simulink model "rtwdemo_symbols"  (Simulink 7.6)
settings: Solver=FixedStepDiscrete  StartTime=0.0  StopTime=1  FixedStep=0.001  RelTol=1e-3
libraries: rtwdemowidgets x1
Description:
  | Identifier Naming Rules
settings Model: Creator=The MathWorks Inc.  ExtModeAutoUpdateStatusClock=off
settings MATStruct: SampleTime=0.001  Offset=0  Priority=[20.0]
settings DataIOCC: SaveOutput=off  SaveTime=off
settings OptimizationCC: InlineParams=on  InlineInvariantSignals=on  PassReuseOutputArgsAs=Individual arguments  StateBitsets=on  DataBitsets=on  UseTempVars=on  ZeroExternalMemoryAtStartup=off  ZeroInternalMemoryAtStartup=off  NoFixptDivByZeroProtection=on  EfficientFloat2IntCast=on  EfficientMapNaN2IntZero=off  OptimizeModelRefInitCode=on  LifeSpan=1  BufferReusableBoundary=off
settings DebuggingCC: CheckExecutionContextPreStartOutputMsg=on  CheckExecutionContextRuntimeOutputMsg=on  SigSpecEnsureSampleTimeMsg=none  StrictBusMsg=ErrorOnBusTreatedAsVector
settings HardwareCC: ProdIntDivRoundTo=Zero  ProdEndianess=LittleEndian  ProdHWDeviceType=Generic->32-bit Embedded Processor  TargetHWDeviceType=Generic->32-bit Embedded Processor
settings SFSimCC: SimParseCustomCode=off
settings RTWCC: SystemTargetFile=ert.tlc  TemplateMakefile=ert_default_tmf  Description=Real-Time Workshop Embedded Coder (no auto configuration)  GenerateReport=on  RTWVerbose=off  ProcessScript=ert_make_rtw_hook  IncludeHyperlinkInReport=on  LaunchReport=on
settings CodeAppCC: ForceParamTrailComments=on  IgnoreCustomStorageClasses=off  IgnoreTestpoints=on  MaxIdLength=40  SimulinkDataObjDesc=on  CustomSymbolStrMacro=$N$M  InsertBlockDesc=on
settings ERTTargetCC: TargetFcnLib=ansi_tfl_tmw.mat  MultiwordLength=2048  GenerateSampleERTMain=on  IncludeMdlTerminateFcn=off  SupportNonFinite=off  SupportComplex=off  InlinedParameterPlacement=NonHierarchical  ERTCustomFileTemplate=example_file_process.tlc  ConvertIfToSwitch=off

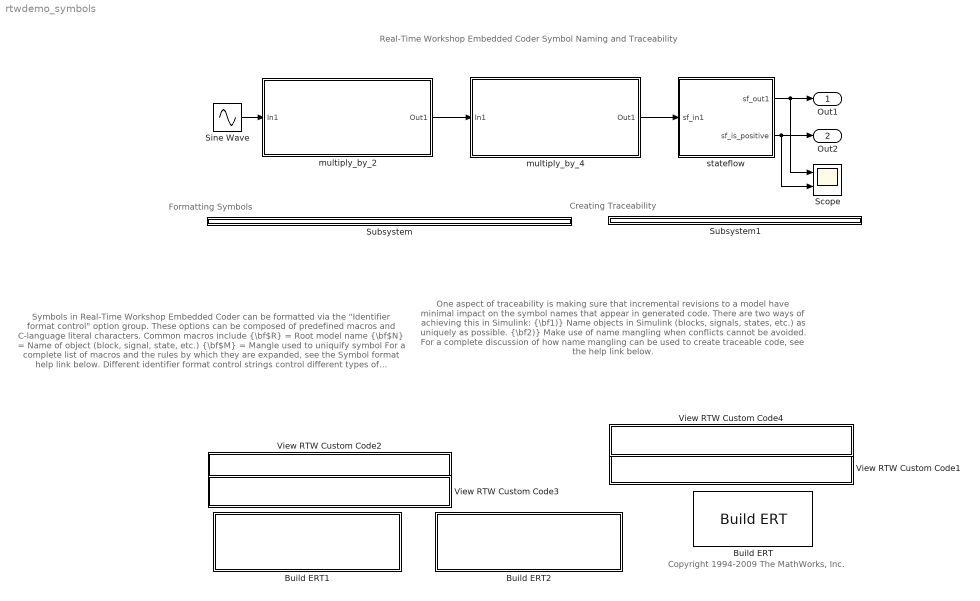
== system rtwdemo_symbols ==
  note: Real-Time Workshop Embedded Coder
      | Symbol Naming and Traceability
  note: Formatting Symbols
  note: Creating Traceability
  note: Symbols in Real-Time Workshop Embedded Coder can be formatted
      | via the "Identifier format control" option group. These options can be
      | composed of predefined macros and C-language literal characters.
      |
      | Common macros include
      |    {\bf$R} = Root model name
      |    {\bf$N} = Name of object (block, signal, state, etc.)
      |    {\bf$M} = Mangle used to uniquify symbol
      |
      | For a complete list of macros and the rules by which they are
      | expanded, see the Symbol format help link below.
      |
      | Different identifier format control strings control different types of identifiers.
      | Double-click the yellow buttons at the bottom to modify the format
      | control strings for global variable names and global type names. Double-
      | click the blue button to generate and inspect code for the change.
  note: One aspect of traceability is making sure that
      | incremental revisions to a model have minimal
      | impact on the symbol names that appear in
      | generated code.  There are two ways of
      | achieving this in Simulink:
      |
      |   {\bf1)} Name objects in Simulink (blocks, signals,
      |        states, etc.) as uniquely as possible.
      |   {\bf2)} Make use of name mangling when conflicts
      |        cannot be avoided.
      |
      | For a complete discussion of how name mangling
      | can be used to create traceable code, see the help
      | link below.
  note: Copyright 1994-2009 The MathWorks, Inc.
  Build ERT : rtwdemowidgets/Build ERT  SystemSampleTime=-1  attrib_overrides={'CustomSymbolStrGlobalVar', 'CustomSymbolStrType','CustomSymbolStrField','CustomSymbolStrFcn','CustomSymbolStrBlkIO','CustomSymbolStrTmpVar','CustomSymbolStrMacro'}
  Build ERT1 : Subsystem  mask{sfs=$R$N$M}
      mask prompts: sfs "symbol format string"
      mask help: Enter the attributes of the configuration set that you want preserved. Otherwise, the default configuration script will override your current settings.
      mask init:
      | if ~isempty(findstr(sfs, '$R'))
      |     dispstr = ['Global variable names\n', ...
      |             'contain model name.\n'];
      | else
      |     dispstr = ['Global variable names do\n',...
      |         'not contain model name.\n'];
      | end
      settings: OpenFcn=|
      | sfs = get_param(bdroot, 'CustomSymbolStrGlobalVar');
      | if strcmp(sfs, '$R$N$M')
      |   sfs = '$N$M';
      | else
      |   sfs = '$R$N$M';
      | end
      | set_param(bdroot, 'CustomSymbolStrGlobalVar', sfs);
      | set_param(gcbh, 'sfs', sfs);  clear sfs;
      mask Display:
      | disp([dispstr,...
      | 	  '(double-click to toggle)'])
  Build ERT2 : Subsystem  mask{sfs=$N$R$M}
      mask prompts: sfs "symbol format string"
      mask help: Enter the attributes of the configuration set that you want preserved. Otherwise, the default configuration script will override your current settings.
      mask init:
      | if ~isempty(findstr(sfs, '$R'))
      |     dispstr = ['Global structure type names\n', ...
      |             'contain model name.\n'];
      | else
      |     dispstr = ['Global structure type names do\n',...
      |         'not contain model name.\n'];
      | end
      settings: OpenFcn=|
      | sfs = get_param(bdroot, 'CustomSymbolStrType');
      | if strcmp(sfs, '$N$R$M')
      |   sfs = '$N$M';
      | else
      |   sfs = '$N$R$M';
      | end
      | set_param(bdroot, 'CustomSymbolStrType', sfs);
      | set_param(gcbh, 'sfs', sfs);   clear sfs;
      mask Display:
      | disp([dispstr,...
      | 	  '(double-click to toggle)'])
  Scope : Scope  NumInputPorts=2
      settings: YMin=-500~0  YMax=500~1
  Sine Wave : Sin  SineType=Sample based  Amplitude=100  SampleTime=.001
  Subsystem : Subsystem
  Subsystem1 : Subsystem
  View RTW Custom Code1 : Subsystem
      mask init:
      | pos    = get_param(gcb, 'Position');
      | width  = pos(3) - pos(1);
      | height = pos(4) - pos(2);
      | 
      | 
      | % Compute arrow coordinates
      | arrowW = width  / 20;
      | arrowH = height / 2.5;
      | arrowX = width  / 50;
      | arrowY = height / 3;
      | arrowXvec = [arrowX, arrowX, arrowX + arrowW];
      | arrowYvec = [arrowY, arrowY + arrowH, arrowY + arrowH / 2];
      | 
      | % Compute text position
      | textXbuff = width / 30;
      | textX  = arrowX + arrowW + textXbuff;
      | textY  = height / 2;
      settings: OpenFcn=helpview([docroot '/toolbox/ecoder/helptargets.map'], 'symbols_traceability')
      mask Display:
      | patch(arrowXvec, arrowYvec);
      | text(textX, textY, 'Double-click to view traceability help');
  View RTW Custom Code2 : Subsystem
      mask init: same as rtwdemo_symbols/View RTW Custom Code1
      settings: OpenFcn=|
      | dlg = slCfgPrmDlg(bdroot,'Open');
      | dlg = slCfgPrmDlg(bdroot,'TurnToPage','Real-Time Workshop/Symbols');clear dlg;
      mask Display:
      | patch(arrowXvec, arrowYvec);
      | text(textX, textY, 'Double-click to view symbol format');
  View RTW Custom Code3 : Subsystem
      mask init: same as rtwdemo_symbols/View RTW Custom Code1
      settings: OpenFcn=helpview([docroot '/toolbox/ecoder/helptargets.map'], 'symbols_pane')
      mask Display:
      | patch(arrowXvec, arrowYvec);
      | text(textX, textY, 'Double-click to view symbol format help');
  View RTW Custom Code4 : Subsystem
      mask init: same as rtwdemo_symbols/View RTW Custom Code1
      settings: OpenFcn=|
      | dlg = slCfgPrmDlg(bdroot,'Open');
      | dlg = slCfgPrmDlg(bdroot,'TurnToPage','Real-Time Workshop/Symbols'); clear dlg;
      mask Display:
      | patch(arrowXvec, arrowYvec);
      | text(textX, textY, 'Double-click to view mangle settings');
  multiply_by_2 : Subsystem  TreatAsAtomicUnit=on
      settings: RTWSystemCode=Function
      mask Display: fprintf('This atomic subsystem will\ngenerate a function of the form\n<model name>_<block name>\nwhich expands to\n%s_%s ',get_param(bdroot(gcbh),'name'),get_param(gcbh,'name'))
  multiply_by_4 : Subsystem  TreatAsAtomicUnit=on
      settings: RTWSystemCode=Function  RTWFcnNameOpts=Use subsystem name
      mask Display: fprintf('This atomic subsystem will\ngenerate a function of the form\n<model name>_<block name>\nwhich expands to\n%s_%s ',get_param(bdroot(gcbh),'name'),get_param(gcbh,'name'))
  stateflow : Stateflow chart  TreatAsAtomicUnit=on
  Out1 : Outport
  Out2 : Outport  Port=2
  wires:
  Sine Wave/1 -> multiply_by_2/1(In1)
  multiply_by_2/1(Out1) -> multiply_by_4/1(In1)
  stateflow/1(sf_out1) -> Out1/1, Scope/1
  multiply_by_4/1(Out1) -> stateflow/1(sf_in1)
  stateflow/2(sf_is_positive) -> Out2/1, Scope/2

== system rtwdemo_symbols/Build ERT1 ==

== system rtwdemo_symbols/Build ERT2 ==

== system rtwdemo_symbols/Subsystem ==

== system rtwdemo_symbols/Subsystem1 ==

== system rtwdemo_symbols/View RTW Custom Code1 ==

== system rtwdemo_symbols/View RTW Custom Code2 ==

== system rtwdemo_symbols/View RTW Custom Code3 ==

== system rtwdemo_symbols/View RTW Custom Code4 ==

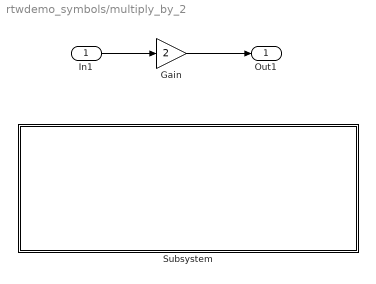
== system rtwdemo_symbols/multiply_by_2 ==
  In1 : Inport
  Gain : Gain  Gain=2
  Subsystem : Subsystem
      settings: OpenFcn=open_system('rtwdemo_symbols/multiply_by_4')
      mask Display: fprintf('The gain block in this subsystem will generate\na symbol named "Gain".  This will collide with\nthe symbol generated for the gain block in\n"rtwdemo_symbols/multiply_by_4/Gain".\n\n (double-click to open colliding block)')
  Out1 : Outport
  wires:
  In1/1 -> Gain/1
  Gain/1 -> Out1/1

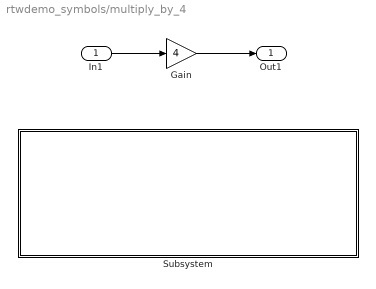
== system rtwdemo_symbols/multiply_by_4 ==
  In1 : Inport
  Gain : Gain  Gain=4
  Subsystem : Subsystem
      settings: OpenFcn=open_system('rtwdemo_symbols/multiply_by_2')
      mask Display: fprintf('The gain block in this subsystem will generate\na symbol named "Gain".  This will collide with\nthe symbol generated for the gain block in\n"rtwdemo_symbols/multiply_by_2/Gain".\n\n (double-click to open colliding block)')
  Out1 : Outport
  wires:
  In1/1 -> Gain/1
  Gain/1 -> Out1/1

== system rtwdemo_symbols/multiply_by_2/Subsystem ==

== system rtwdemo_symbols/multiply_by_4/Subsystem ==

== stateflow chart stateflow ==
  state positive_state
    entry:
    sf_is_positive = 1;
    sf_out1 = sf_in1;
  state negative_state
    entry:
    sf_is_positive = 0;
    sf_out1 = sf_in1;
  state result = sf_is_positive(val) [function]
    (default) -> (junction 7)
    (junction 7) -> (junction 8) [order 1] : [val > 0]
        | {result = 1;}
    (junction 10) -> (junction 9) : {result = 0;}
    (junction 7) -> (junction 10) [order 2]
  note: Note:
      | For demonstration purposes, inlining has been
      | turned off for this graphical function.  As a result,
      | a separate c-code function will be generated that
      | respects the Real-Time Workshop naming rules.
  (default) -> positive_state
  positive_state -> negative_state : [~sf_is_positive(sf_in1)]
  negative_state -> positive_state : [sf_is_positive(sf_in1)]
  data: result function_output double; val function_input double; sf_in1 input double; sf_out1 output double; sf_is_positive output double
